simulink model "CalcSpinSpeednDir"  (R2020b)
settings: Solver=FixedStepDiscrete  StartTime=0.0  StopTime=100  FixedStep=0.0002  RelTol=1e-3
values from neighbouring files (symbols this model uses):
  p = 8/2    (= 4)    [MotorControlLibData.m]    (also in local_pmsm_torque_control_data.m = 8)
  Ts = 250.0e-06    (= 0.00025)    [MotorControlLibData.m]    (also in local_pmsm_torque_control_data.m = 5e-06)
libraries: simulink x6
settings Model: DataDictionary=CalcSpeednDir.sldd  Creator=unix  LastModifiedBy=unix
settings SolverCC: AutoInsertRateTranBlk=on
settings DataIOCC: SaveOutput=off  SaveTime=off
settings OptimizationCC: DefaultParameterBehavior=Inlined  EnhancedBackFolding=on  PassReuseOutputArgsAs=Individual arguments  ZeroExternalMemoryAtStartup=off  ZeroInternalMemoryAtStartup=off  OptimizeBlockOrder=speed  DifferentSizesBufferReuse=on  OptimizationCustomize=off  EfficientTunableParamExpr=on
settings DebuggingCC: SignalInfNanChecking=warning  SignalRangeChecking=warning  CheckMatrixSingularityMsg=warning  IntegerOverflowMsg=error  ParameterOverflowMsg=warning  ParameterUnderflowMsg=warning  ParameterPrecisionLossMsg=none  ParameterTunabilityLossMsg=error  UnderSpecifiedDataTypeMsg=warning  IntegerSaturationMsg=error
settings SFSimCC: MATLABDynamicMemAlloc=off
settings RTWCC: Description=Embedded Coder  SystemTargetFile=ert.tlc  GenCodeOnly=on  TemplateMakefile=ert_default_tmf  GenerateReport=on  IncludeHyperlinkInReport=on  LaunchReport=on  GenerateTraceInfo=on  GenerateTraceReport=on  GenerateTraceReportSl=on  GenerateTraceReportSf=on  GenerateTraceReportEml=on
settings CodeAppCC: ForceParamTrailComments=on  IgnoreCustomStorageClasses=off  OperatorAnnotations=on  SimulinkDataObjDesc=on  SFDataObjDesc=on  InsertBlockDesc=on
settings ERTTargetCC: TargetLangStandard=C99 (ISO)  GenerateSampleERTMain=on  GenerateASAP2=on  InlinedParameterPlacement=NonHierarchical  ERTCustomFileTemplate=example_file_process.tlc

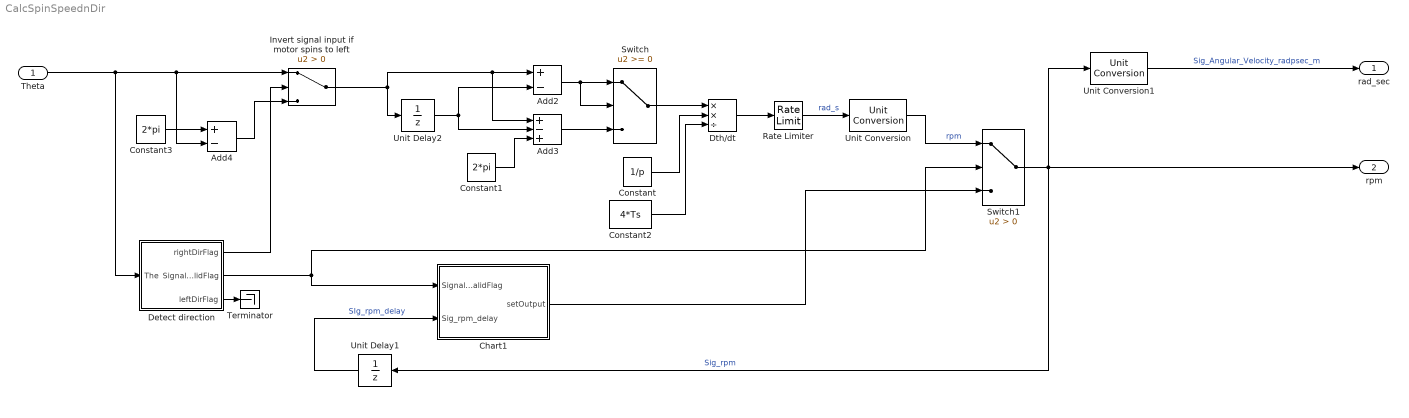
== system CalcSpinSpeednDir ==
  Theta : Inport  OutDataTypeStr=single  PortDimensions=1  SampleTime=[0.00020000000000000001,0]
  Add2 : Sum  Inputs=+-
  Add3 : Sum  Inputs=+-+
  Add4 : Sum  Inputs=+-
  Chart1 : Stateflow chart  TreatAsAtomicUnit=on
  Constant : Constant  Value=1/p  OutDataTypeStr=single
  Constant1 : Constant  Value=2*pi  OutDataTypeStr=single
  Constant2 : Constant  Value=4*Ts  OutDataTypeStr=single
  Constant3 : Constant  Value=2*pi  OutDataTypeStr=Inherit: Inherit via back propagation
  "Detect direction " : Subsystem
  Dth/dt : Product  Inputs=**/
  Invert signal input if motor spins to left : Switch  Criteria=u2 > Threshold
  Rate Limiter : RateLimiter  RisingSlewLimit=50000  FallingSlewLimit=-50000  SampleTimeMode=inherited
  Switch : Switch  OutDataTypeStr=single
  Switch1 : Switch  Criteria=u2 > Threshold  OutDataTypeStr=single
  Terminator : Terminator
  Unit Conversion : UnitConversion
  Unit Conversion1 : UnitConversion  OutputType=Inherit: Inherit via back propagation
  Unit Delay1 : UnitDelay  SampleTime=-1  HasFrameUpgradeWarning=on
  Unit Delay2 : UnitDelay  SampleTime=-1  HasFrameUpgradeWarning=on
  rad_sec : Outport  OutDataTypeStr=single  Unit=rad/sec  PortDimensions=1  SampleTime=[0.00020000000000000001,0]
  rpm : Outport  Port=2  OutDataTypeStr=single  Unit=rpm  PortDimensions=1  SampleTime=[0.00020000000000000001,0]
  wires:
  Rate Limiter/1 -> Unit Conversion/1  "rad_s"
  Add3/1 -> Switch/3
  Unit Delay2/1 -> Add2/2, Add3/2
  Switch/1 -> Dth/dt/1
  Add2/1 -> Switch/1, Switch/2
  Constant1/1 -> Add3/3
  Constant/1 -> Dth/dt/2
  "Detect direction "/1(rightDirFlag) -> Invert signal input if motor spins to left/2
  Constant3/1 -> Add4/1
  Theta/1 -> "Detect direction "/1(The), Invert signal input if motor spins to left/1, Add4/2
  Add4/1 -> Invert signal input if motor spins to left/3
  Invert signal input if motor spins to left/1 -> Add2/1, Add3/1, Unit Delay2/1
  "Detect direction "/3(leftDirFlag) -> Terminator/1
  "Detect direction "/2(SignalValidFlag) -> Chart1/1(SignalValidFlag), Switch1/2
  Unit Delay1/1 -> Chart1/2(Sig_rpm_delay)  "SIg_rpm_delay"
  Switch1/1 -> Unit Conversion1/1, rpm/1, Unit Delay1/1  "Sig_rpm"
  Chart1/1(setOutput) -> Switch1/3
  Unit Conversion/1 -> Switch1/1  "rpm"
  Unit Conversion1/1 -> rad_sec/1  "Sig_Angular_Velocity_radpsec_m"
  Constant2/1 -> Dth/dt/3
  Dth/dt/1 -> Rate Limiter/1

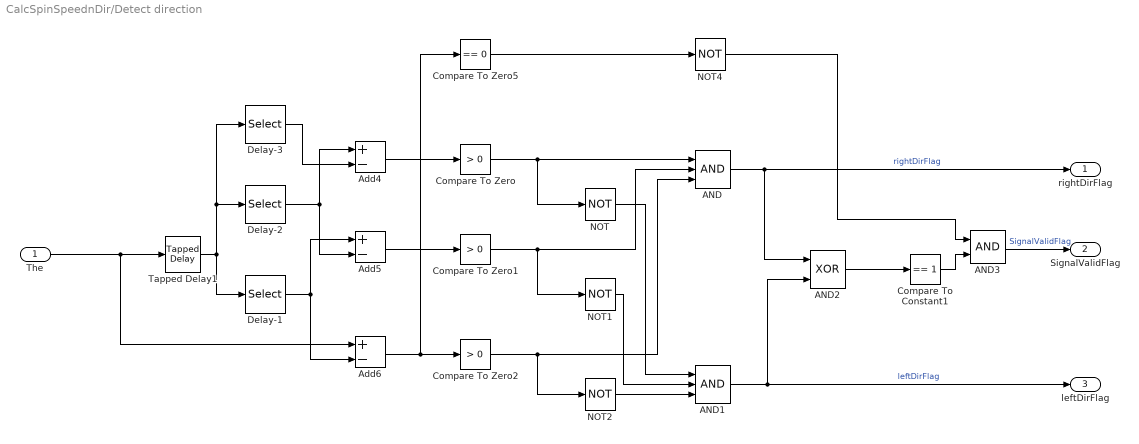
== system CalcSpinSpeednDir/Detect direction  ==
  The : Inport
  AND : Logic  Inputs=3  AllPortsSameDT=off  OutDataTypeStr=boolean
  AND1 : Logic  Inputs=3  AllPortsSameDT=off  OutDataTypeStr=boolean
  AND2 : Logic  Operator=XOR  AllPortsSameDT=off  OutDataTypeStr=boolean
  AND3 : Logic  AllPortsSameDT=off  OutDataTypeStr=boolean
  Add4 : Sum  Inputs=+-
  Add5 : Sum  Inputs=+-
  Add6 : Sum  Inputs=+-
  Compare To Constant1 : simulink/Logic and Bit Operations/Compare To Constant  relop===  const=1  OutDataTypeStr=boolean
  Compare To Zero : simulink/Logic and Bit Operations/Compare To Zero  relop=>  OutDataTypeStr=boolean
  Compare To Zero1 : simulink/Logic and Bit Operations/Compare To Zero  relop=>  OutDataTypeStr=boolean
  Compare To Zero2 : simulink/Logic and Bit Operations/Compare To Zero  relop=>  OutDataTypeStr=boolean
  Compare To Zero5 : simulink/Logic and Bit Operations/Compare To Zero  relop===  OutDataTypeStr=boolean
  Delay-1 : Selector  InputPortWidth=3  IndexOptions=Index vector (dialog)  Indices=3  OutputSizes=1
  Delay-2 : Selector  InputPortWidth=3  IndexOptions=Index vector (dialog)  Indices=2  OutputSizes=1
  Delay-3 : Selector  InputPortWidth=3  IndexOptions=Index vector (dialog)  Indices=1  OutputSizes=1
  NOT{,1..2,4} (4 alike) : Logic  Operator=NOT  IconShape=distinctive  AllPortsSameDT=off  OutDataTypeStr=boolean
  Tapped Delay1 : simulink/Discrete/Tapped Delay  vinit=0.0  samptime=-1  NumDelays=3  DelayOrder=Oldest  includeCurrent=off
  rightDirFlag : Outport
  SignalValidFlag : Outport  Port=2
  leftDirFlag : Outport  Port=3
  wires:
  Compare To Constant1/1 -> AND3/2
  NOT4/1 -> AND3/1
  Compare To Zero5/1 -> NOT4/1
  AND2/1 -> Compare To Constant1/1
  AND3/1 -> SignalValidFlag/1  "SignalValidFlag"
  Compare To Zero1/1 -> AND/2, NOT1/1
  The/1 -> Add6/1, Tapped Delay1/1
  NOT2/1 -> AND1/3
  NOT/1 -> AND1/1
  Tapped Delay1/1 -> Delay-3/1, Delay-2/1, Delay-1/1
  Compare To Zero/1 -> NOT/1, AND/1
  Delay-2/1 -> Add5/2, Add4/1
  AND/1 -> AND2/1, rightDirFlag/1  "rightDirFlag"
  AND1/1 -> AND2/2, leftDirFlag/1  "leftDirFlag"
  Add5/1 -> Compare To Zero1/1
  Add6/1 -> Compare To Zero2/1, Compare To Zero5/1
  NOT1/1 -> AND1/2
  Compare To Zero2/1 -> AND/3, NOT2/1
  Delay-3/1 -> Add4/2
  Delay-1/1 -> Add6/2, Add5/1
  Add4/1 -> Compare To Zero/1

== stateflow chart CalcSpinSpeednDir/Chart1 ==
  state InvalidSignal
    en:count = count + 1;
    state noTimeout
      du:count++;
      state MotorWasInRotation
        en:setOutput=Sig_rpm_delay;
        du:setOutput=Sig_rpm_delay;
      state MotorWasStalled
        en:setOutput=0;
        du:setOutput=0;
      (default) -> (junction 60)
      (junction 60) -> MotorWasStalled [order 2]
      (junction 60) -> MotorWasInRotation [order 1] : [Sig_rpm_delay!=0]
    state timeout
      en:setOutput=0;
    (default) -> noTimeout
    noTimeout -> timeout : [count>3]
  state ValidSignal1
    du:count = 0;
  (default) -> (junction 48)
  (junction 48) -> ValidSignal1 [order 2]
  (junction 48) -> InvalidSignal [order 1] : [SignalValidFlag==0]
  InvalidSignal -> ValidSignal1 : [SignalValidFlag==1]
  ValidSignal1 -> InvalidSignal : [SignalValidFlag==0]
  data: SignalValidFlag input; Sig_rpm_delay input; count local uint8; setOutput output double
